simulink model "CANBlocksTemplate"  (Simulink 10.0)
settings: Solver=ode45  StartTime=0.0  StopTime=10.0  RelTol=1e-3  EnableMultiTasking=on
undefined symbols (not defined in the file): IO_Blk_Lib_TTC500, IO_Blk_Lib_TTC9094, IO_CAN_ConfigMsg, IO_CAN_Init, IO_CAN_ReadMsg
libraries: simulink x19, IOBlock_Library_TTC580 x18
(part 2 of 2)

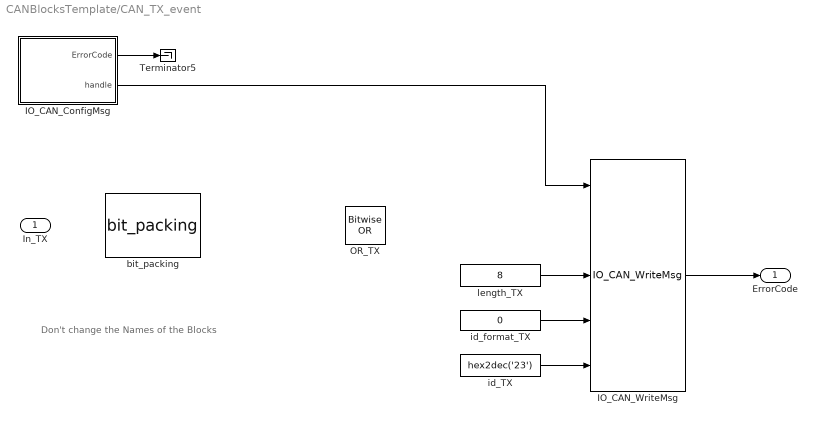
== system CANBlocksTemplate/CAN_TX_event ==
  note: Don't change the Names of the Blocks
  In_TX : Inport
  IO_CAN_ConfigMsg : Subsystem  mask(IO_CAN_ConfigMsg_Code){SampleTime=-1, ttlib=IO_Blk_Lib_TTC500, ttDescription=IO_CAN_ConfigMsg, tt_iolib_version=0.19, channel=IO_CAN_CHANNEL_0, mode=IO_CAN_MSG_READ, id_format=IO_CAN_STD_FRAME, id=0x1, ac_mask=0x7FF}
      mask help: Configures a message object for the given CAN channel.
      mask init:
      | %
      settings: CopyFcn=%deleted
      mask Help: web(which('IO_CAN.h'))
      mask TypeOptions channel: IO_CAN_CHANNEL_0  | IO_CAN_CHANNEL_1 | IO_CAN_CHANNEL_2 | IO_CAN_CHANNEL_3 | IO_CAN_CHANNEL_4 | IO_CAN_CHANNEL_5 | IO_CAN_CHANNEL_6
      mask Callback channel: %
      mask TypeOptions mode: IO_CAN_MSG_READ | IO_CAN_MSG_WRITE
      mask Callback mode: %
      mask TypeOptions id_format: IO_CAN_STD_FRAME | IO_CAN_EXT_FRAME
      mask Callback id_format: %
      mask Callback id: %
      mask Callback ac_mask: %
  IO_CAN_WriteMsg : IOBlock_Library_TTC580/CAN  Blocks TTC580 IOlib/WriteMsg_CAN/IO_CAN_WriteMsg  SampleTime=-1  ttlib=IO_Blk_Lib_TTC500  ttDescription=IO_CAN_WriteMsg  tt_iolib_version=0.19
      settings: SourceProductName=I/O Blocklibrary for TTC580
  OR_TX : simulink/Logic and Bit Operations/Bitwise Operator  logicop=OR  UseBitMask=off  BitMask=bin2dec('11011001')  BitMaskRealWorld=Stored Integer
  Terminator5 : Terminator
  bit_packing : IOBlock_Library_TTC580/CAN  Blocks TTC580 IOlib/bit_packing  SampleTime=-1  ttlib=IO_Blk_Lib_TTC500  ttDescription=bit_packing  tt_iolib_version=0.26  Endianness=little  Format=unsigned  Inversion=off  Startbit=0  Width_bits=8  Factor=1.0  Offset=0.0
      settings: SourceProductName=I/O Blocklibrary for TTC580
  id_TX : Constant  Value=hex2dec('23')  OutDataTypeStr=uint32
  id_format_TX : Constant  Value=0  OutDataTypeStr=Inherit: Inherit via back propagation
  length_TX : Constant  Value=8  OutDataTypeStr=Inherit: Inherit via back propagation
  ErrorCode : Outport  VectorParamsAs1DForOutWhenUnconnected=off
  wires:
  IO_CAN_WriteMsg/1 -> ErrorCode/1
  IO_CAN_ConfigMsg/1(ErrorCode) -> Terminator5/1
  IO_CAN_ConfigMsg/2(handle) -> IO_CAN_WriteMsg/1
  length_TX/1 -> IO_CAN_WriteMsg/3
  id_format_TX/1 -> IO_CAN_WriteMsg/4
  id_TX/1 -> IO_CAN_WriteMsg/5

== system CANBlocksTemplate/Config_CAN_Tx_aggregate ==
  note: Use this in case DBC_Import()
      | was called with AggegationCycleLimit
      | set to smaller or equal of actual
      | CycleTime according do dbc-file
  IO_CAN_ConfigMsg : Subsystem  mask(IO_CAN_ConfigMsg_Code){SampleTime=-1, ttlib=IO_Blk_Lib_TTC500, ttDescription=IO_CAN_ConfigMsg, tt_iolib_version=0.19, channel=IO_CAN_CHANNEL_0, mode=IO_CAN_MSG_READ, id_format=IO_CAN_STD_FRAME, id=0x1, ac_mask=0x7FF}
      mask help: Configures a message object for the given CAN channel.
      mask init:
      | %
      settings: CopyFcn=%deleted
      mask Help: web(which('IO_CAN.h'))
      mask TypeOptions channel: IO_CAN_CHANNEL_0  | IO_CAN_CHANNEL_1 | IO_CAN_CHANNEL_2 | IO_CAN_CHANNEL_3 | IO_CAN_CHANNEL_4 | IO_CAN_CHANNEL_5 | IO_CAN_CHANNEL_6
      mask Callback channel: %
      mask TypeOptions mode: IO_CAN_MSG_READ | IO_CAN_MSG_WRITE
      mask Callback mode: %
      mask TypeOptions id_format: IO_CAN_STD_FRAME | IO_CAN_EXT_FRAME
      mask Callback id_format: %
      mask Callback id: %
      mask Callback ac_mask: %
  Terminator5 : Terminator
  tag scope: A=global
  wires:
  IO_CAN_ConfigMsg/2(handle) -> [A]
  IO_CAN_ConfigMsg/1(ErrorCode) -> Terminator5/1

== system CANBlocksTemplate/IO_CAN_Init ==
  Constant : Constant  Value=0  OutDataTypeStr=uint16
  ErrorCode : Outport  VectorParamsAs1DForOutWhenUnconnected=off
  wires:
  Constant/1 -> ErrorCode/1

== system CANBlocksTemplate/CAN_RX/IO_CAN_ConfigMsg ==
  IO_CAN_ConfigMsg_s : S-Function  FunctionName=IO_CAN_ConfigMsg_s  Parameters=SampleTime,channel,mode,id_format,id,ac_mask  SFunctionDeploymentMode=off  EnableBusSupport=off
  ErrorCode : Outport  VectorParamsAs1DForOutWhenUnconnected=off
  handle : Outport  Port=2  VectorParamsAs1DForOutWhenUnconnected=off
  wires:
  IO_CAN_ConfigMsg_s/2 -> handle/1
  IO_CAN_ConfigMsg_s/1 -> ErrorCode/1

== system CANBlocksTemplate/CAN_RX/Trigger_Block ==
  Compare To Constant : simulink/Logic and Bit Operations/Compare To Constant  relop===  const=trigger_offset  OutDataTypeStr=boolean  ZeroCross=off
  Counter Limited : simulink/Sources/Counter Limited  uplimit=max(derate - 1,0)  tsamp=-1
  Trigger : Outport  VectorParamsAs1DForOutWhenUnconnected=off
  wires:
  Counter Limited/1 -> Compare To Constant/1
  Compare To Constant/1 -> Trigger/1

== system CANBlocksTemplate/CAN_RX_ND/IO_CAN_ConfigMsg ==
  IO_CAN_ConfigMsg_s : S-Function  FunctionName=IO_CAN_ConfigMsg_s  Parameters=SampleTime,channel,mode,id_format,id,ac_mask  SFunctionDeploymentMode=off  EnableBusSupport=off
  ErrorCode : Outport  VectorParamsAs1DForOutWhenUnconnected=off
  handle : Outport  Port=2  VectorParamsAs1DForOutWhenUnconnected=off
  wires:
  IO_CAN_ConfigMsg_s/1 -> ErrorCode/1
  IO_CAN_ConfigMsg_s/2 -> handle/1

== system CANBlocksTemplate/CAN_RX_ND/IO_CAN_ReadMsg ==
  handle : Inport
  Enable : EnablePort
  IO_CAN_ReadMsg : IOBlock_Library_TTC580/CAN  Blocks TTC580 IOlib/ReadMsg_CAN/IO_CAN_ReadMsg  SampleTime=-1  ttlib=IO_Blk_Lib_TTC500  ttDescription=IO_CAN_ReadMsg  tt_iolib_version=0.19
      settings: SourceProductName=I/O Blocklibrary for TTC580
  ErrorCode : Outport  VectorParamsAs1DForOutWhenUnconnected=off
  buffer_data : Outport  Port=2  VectorParamsAs1DForOutWhenUnconnected=off
  buffer_length : Outport  Port=3  VectorParamsAs1DForOutWhenUnconnected=off
  buffer_id_format : Outport  Port=4  VectorParamsAs1DForOutWhenUnconnected=off
  buffer_id : Outport  Port=5  VectorParamsAs1DForOutWhenUnconnected=off
  wires:
  handle/1 -> IO_CAN_ReadMsg/1
  IO_CAN_ReadMsg/1 -> ErrorCode/1
  IO_CAN_ReadMsg/2 -> buffer_data/1
  IO_CAN_ReadMsg/3 -> buffer_length/1
  IO_CAN_ReadMsg/4 -> buffer_id_format/1
  IO_CAN_ReadMsg/5 -> buffer_id/1

== system CANBlocksTemplate/CAN_RX_ND/Trigger_Block ==
  Compare To Constant : simulink/Logic and Bit Operations/Compare To Constant  relop===  const=trigger_offset  OutDataTypeStr=boolean  ZeroCross=off
  Counter Limited : simulink/Sources/Counter Limited  uplimit=max(derate - 1,0)  tsamp=-1
  Trigger : Outport  VectorParamsAs1DForOutWhenUnconnected=off
  wires:
  Counter Limited/1 -> Compare To Constant/1
  Compare To Constant/1 -> Trigger/1

== system CANBlocksTemplate/CAN_RX_NONE/IO_CAN_ConfigMsg ==
  IO_CAN_ConfigMsg_s : S-Function  FunctionName=IO_CAN_ConfigMsg_s  Parameters=SampleTime,channel,mode,id_format,id,ac_mask  SFunctionDeploymentMode=off  EnableBusSupport=off
  ErrorCode : Outport  VectorParamsAs1DForOutWhenUnconnected=off
  handle : Outport  Port=2  VectorParamsAs1DForOutWhenUnconnected=off
  wires:
  IO_CAN_ConfigMsg_s/2 -> handle/1
  IO_CAN_ConfigMsg_s/1 -> ErrorCode/1

== system CANBlocksTemplate/CAN_RX_NONE/Trigger_Block ==
  Compare To Constant : simulink/Logic and Bit Operations/Compare To Constant  relop===  const=trigger_offset  OutDataTypeStr=boolean  ZeroCross=off
  Counter Limited : simulink/Sources/Counter Limited  uplimit=max(derate - 1,0)  tsamp=-1
  Trigger : Outport  VectorParamsAs1DForOutWhenUnconnected=off
  wires:
  Counter Limited/1 -> Compare To Constant/1
  Compare To Constant/1 -> Trigger/1

== system CANBlocksTemplate/CAN_RX_NONE_ND/IO_CAN_ConfigMsg ==
  IO_CAN_ConfigMsg_s : S-Function  FunctionName=IO_CAN_ConfigMsg_s  Parameters=SampleTime,channel,mode,id_format,id,ac_mask  SFunctionDeploymentMode=off  EnableBusSupport=off
  ErrorCode : Outport  VectorParamsAs1DForOutWhenUnconnected=off
  handle : Outport  Port=2  VectorParamsAs1DForOutWhenUnconnected=off
  wires:
  IO_CAN_ConfigMsg_s/1 -> ErrorCode/1
  IO_CAN_ConfigMsg_s/2 -> handle/1

== system CANBlocksTemplate/CAN_RX_NONE_ND/IO_CAN_ReadMsg ==
  handle : Inport
  Enable : EnablePort
  IO_CAN_ReadMsg : IOBlock_Library_TTC580/CAN  Blocks TTC580 IOlib/ReadMsg_CAN/IO_CAN_ReadMsg  SampleTime=-1  ttlib=IO_Blk_Lib_TTC500  ttDescription=IO_CAN_ReadMsg  tt_iolib_version=0.19
      settings: SourceProductName=I/O Blocklibrary for TTC580
  ErrorCode : Outport  VectorParamsAs1DForOutWhenUnconnected=off
  buffer_data : Outport  Port=2  VectorParamsAs1DForOutWhenUnconnected=off
  buffer_length : Outport  Port=3  VectorParamsAs1DForOutWhenUnconnected=off
  buffer_id_format : Outport  Port=4  VectorParamsAs1DForOutWhenUnconnected=off
  buffer_id : Outport  Port=5  VectorParamsAs1DForOutWhenUnconnected=off
  wires:
  handle/1 -> IO_CAN_ReadMsg/1
  IO_CAN_ReadMsg/1 -> ErrorCode/1
  IO_CAN_ReadMsg/2 -> buffer_data/1
  IO_CAN_ReadMsg/3 -> buffer_length/1
  IO_CAN_ReadMsg/4 -> buffer_id_format/1
  IO_CAN_ReadMsg/5 -> buffer_id/1

== system CANBlocksTemplate/CAN_RX_NONE_ND/Trigger_Block ==
  Compare To Constant : simulink/Logic and Bit Operations/Compare To Constant  relop===  const=trigger_offset  OutDataTypeStr=boolean  ZeroCross=off
  Counter Limited : simulink/Sources/Counter Limited  uplimit=max(derate - 1,0)  tsamp=-1
  Trigger : Outport  VectorParamsAs1DForOutWhenUnconnected=off
  wires:
  Counter Limited/1 -> Compare To Constant/1
  Compare To Constant/1 -> Trigger/1

== system CANBlocksTemplate/CAN_RX_NONE_event/IO_CAN_ConfigMsg ==
  IO_CAN_ConfigMsg_s : S-Function  FunctionName=IO_CAN_ConfigMsg_s  Parameters=SampleTime,channel,mode,id_format,id,ac_mask  SFunctionDeploymentMode=off  EnableBusSupport=off
  ErrorCode : Outport  VectorParamsAs1DForOutWhenUnconnected=off
  handle : Outport  Port=2  VectorParamsAs1DForOutWhenUnconnected=off
  wires:
  IO_CAN_ConfigMsg_s/1 -> ErrorCode/1
  IO_CAN_ConfigMsg_s/2 -> handle/1

== system CANBlocksTemplate/CAN_RX_event/IO_CAN_ConfigMsg ==
  IO_CAN_ConfigMsg_s : S-Function  FunctionName=IO_CAN_ConfigMsg_s  Parameters=SampleTime,channel,mode,id_format,id,ac_mask  SFunctionDeploymentMode=off  EnableBusSupport=off
  ErrorCode : Outport  VectorParamsAs1DForOutWhenUnconnected=off
  handle : Outport  Port=2  VectorParamsAs1DForOutWhenUnconnected=off
  wires:
  IO_CAN_ConfigMsg_s/1 -> ErrorCode/1
  IO_CAN_ConfigMsg_s/2 -> handle/1

== system CANBlocksTemplate/CAN_TX/IO_CAN_ConfigMsg ==
  IO_CAN_ConfigMsg_s : S-Function  FunctionName=IO_CAN_ConfigMsg_s  Parameters=SampleTime,channel,mode,id_format,id,ac_mask  SFunctionDeploymentMode=off  EnableBusSupport=off
  ErrorCode : Outport  VectorParamsAs1DForOutWhenUnconnected=off
  handle : Outport  Port=2  VectorParamsAs1DForOutWhenUnconnected=off
  wires:
  IO_CAN_ConfigMsg_s/2 -> handle/1
  IO_CAN_ConfigMsg_s/1 -> ErrorCode/1

== system CANBlocksTemplate/CAN_TX/Trigger_Block ==
  Compare To Constant : simulink/Logic and Bit Operations/Compare To Constant  relop===  const=trigger_offset  OutDataTypeStr=boolean  ZeroCross=off
  Counter Limited : simulink/Sources/Counter Limited  uplimit=max(derate - 1,0)  tsamp=-1
  Trigger : Outport  VectorParamsAs1DForOutWhenUnconnected=off
  wires:
  Counter Limited/1 -> Compare To Constant/1
  Compare To Constant/1 -> Trigger/1

== system CANBlocksTemplate/CAN_TX_NONE/IO_CAN_ConfigMsg ==
  IO_CAN_ConfigMsg_s : S-Function  FunctionName=IO_CAN_ConfigMsg_s  Parameters=SampleTime,channel,mode,id_format,id,ac_mask  SFunctionDeploymentMode=off  EnableBusSupport=off
  ErrorCode : Outport  VectorParamsAs1DForOutWhenUnconnected=off
  handle : Outport  Port=2  VectorParamsAs1DForOutWhenUnconnected=off
  wires:
  IO_CAN_ConfigMsg_s/2 -> handle/1
  IO_CAN_ConfigMsg_s/1 -> ErrorCode/1

== system CANBlocksTemplate/CAN_TX_NONE/Trigger_Block ==
  Compare To Constant : simulink/Logic and Bit Operations/Compare To Constant  relop===  const=trigger_offset  OutDataTypeStr=boolean  ZeroCross=off
  Counter Limited : simulink/Sources/Counter Limited  uplimit=max(derate - 1,0)  tsamp=-1
  Trigger : Outport  VectorParamsAs1DForOutWhenUnconnected=off
  wires:
  Counter Limited/1 -> Compare To Constant/1
  Compare To Constant/1 -> Trigger/1

== system CANBlocksTemplate/CAN_TX_NONE_aggr/Trigger_Block ==
  Compare To Constant : simulink/Logic and Bit Operations/Compare To Constant  relop===  const=trigger_offset  OutDataTypeStr=boolean  ZeroCross=off
  Counter Limited : simulink/Sources/Counter Limited  uplimit=max(derate - 1,0)  tsamp=-1
  Trigger : Outport  VectorParamsAs1DForOutWhenUnconnected=off
  wires:
  Compare To Constant/1 -> Trigger/1
  Counter Limited/1 -> Compare To Constant/1

== system CANBlocksTemplate/CAN_TX_NONE_event/IO_CAN_ConfigMsg ==
  IO_CAN_ConfigMsg_s : S-Function  FunctionName=IO_CAN_ConfigMsg_s  Parameters=SampleTime,channel,mode,id_format,id,ac_mask  SFunctionDeploymentMode=off  EnableBusSupport=off
  ErrorCode : Outport  VectorParamsAs1DForOutWhenUnconnected=off
  handle : Outport  Port=2  VectorParamsAs1DForOutWhenUnconnected=off
  wires:
  IO_CAN_ConfigMsg_s/1 -> ErrorCode/1
  IO_CAN_ConfigMsg_s/2 -> handle/1

== system CANBlocksTemplate/CAN_TX_aggr/Trigger_Block ==
  Compare To Constant : simulink/Logic and Bit Operations/Compare To Constant  relop===  const=trigger_offset  OutDataTypeStr=boolean  ZeroCross=off
  Counter Limited : simulink/Sources/Counter Limited  uplimit=max(derate - 1,0)  tsamp=-1
  Trigger : Outport  VectorParamsAs1DForOutWhenUnconnected=off
  wires:
  Counter Limited/1 -> Compare To Constant/1
  Compare To Constant/1 -> Trigger/1

== system CANBlocksTemplate/CAN_TX_event/IO_CAN_ConfigMsg ==
  IO_CAN_ConfigMsg_s : S-Function  FunctionName=IO_CAN_ConfigMsg_s  Parameters=SampleTime,channel,mode,id_format,id,ac_mask  SFunctionDeploymentMode=off  EnableBusSupport=off
  ErrorCode : Outport  VectorParamsAs1DForOutWhenUnconnected=off
  handle : Outport  Port=2  VectorParamsAs1DForOutWhenUnconnected=off
  wires:
  IO_CAN_ConfigMsg_s/1 -> ErrorCode/1
  IO_CAN_ConfigMsg_s/2 -> handle/1

== system CANBlocksTemplate/Config_CAN_Tx_aggregate/IO_CAN_ConfigMsg ==
  IO_CAN_ConfigMsg_s : S-Function  FunctionName=IO_CAN_ConfigMsg_s  Parameters=SampleTime,channel,mode,id_format,id,ac_mask  SFunctionDeploymentMode=off  EnableBusSupport=off
  ErrorCode : Outport  VectorParamsAs1DForOutWhenUnconnected=off
  handle : Outport  Port=2  VectorParamsAs1DForOutWhenUnconnected=off
  wires:
  IO_CAN_ConfigMsg_s/2 -> handle/1
  IO_CAN_ConfigMsg_s/1 -> ErrorCode/1
